simulink model "proprioception_test"  (R2015a)
settings: Solver=ode4  SolverMode=MultiTasking  StartTime=0.0  StopTime=inf  FixedStep=BKIN_STEP_TIME  RelTol=1e-3
StartFcn:
  |  warndlg('Dexterit-E models cannot run under simulation. Please compile your model and run it from within Dexterit-E.');set_param(bdroot,'SimulationCommand','stop')
model workspace (MAT data in the model file):
  col_x = 1
  col_y = 2
  RADIUS_VIS = 3
  COLOR_INIT = 4
  DELAY_POST_TRIAL_COL = 5
  BKIN_STEP_TIME = 0.00025
  COLOR_MOVE = 5
  START_WAIT_TIME_COL = 1
  E_START_TRIAL = 2
  E_START_REACHED = 4
  E_MOVED_EARLY = 21
  E_GO_CUE = 9
  E_MOVE_TIMEOUT = 23
  E_HOLDING_STILL = 12
  E_END_TRIAL = 14
  STROKE_WIDTH = 6
  K_HAND_VEL = 1
  E_MOVE_ON = 10
  K_HOLDTIME = 2
  K_ROBOT_RAMP_TIME = 3
  E_ROBOT_RETURN_TO_START = 33
  E_ENABLED_CONTROLLER = 31
  K_TIME_TO_START = 4
  E_RETURN_TO_START = 35
  E_HOLD_POS = 37
  E_INCREMENTING_TSTEP1 = 6
  E_INCREMENTING_TSTEP2 = 7
  E_INCREMENTING_TSTEP3 = 8
  BKIN_KINEMATIC_FRAME_SIZE = 400
  E_NO_EVENT = 0
  COMP_IS_SAME = 2
  E_QUESTION1 = 40
  REFERENCE_TGT = 6
  CP1 = 7
  CP2 = 8
  CP3 = 9
  CP4 = 10
  MOVE_TO_REF_TIME = 2
  REPOSITION_TIME = 3
  STARTUP_TIME = 4
  COMP_IS_DIFF = 3
  ROTATION = 7
  E_WAIT_JS_THRESH = 16
  E_AT_JS_THRESH = 18
libraries: simulink x5, Video x4, General x3, slrtlib x3, KINARM_loads x2, KINARM_IO x1, KINARM_general x1, xpcnilib x1
CloseFcn:
  | rtwprivate ssgencode ModelCloseRequest b2lab2d
settings Model: ModifiedComment=chris -- Wed Feb 16 09:18:30 2005 -- Version 1.1384  ModifiedHistory=Feb 16/05 - Add error repeat, add offset ramp  ExtModeArmWhenConnect=off  ExtModeLogAll=off  Creator=Chris Grebeldinger  LastModifiedBy=User
settings SolverCC: EnableConcurrentExecution=on  AutoInsertRateTranBlk=on
settings DataIOCC: LimitDataPoints=off  SignalLoggingSaveFormat=ModelDataLogs  SaveOutput=off  SaveTime=off  SignalLoggingName=sigsOut
settings OptimizationCC: BlockReduction=off  BooleanDataType=off  OptimizeBlockIOStorage=off  BufferReuse=off  GlobalBufferReuse=off  ExpressionFolding=off  ExpressionDepthLimit=2147483647  LocalBlockOutputs=off  InitFltsAndDblsToZero=on
settings DebuggingCC: SaveWithParameterizedLinksMsg=none  UnderspecifiedInitializationDetection=Classic  MergeDetectMultiDrivingBlocksExec=none  SignalResolutionControl=TryResolveAllWithWarning  MultiTaskDSMMsg=warning  FcnCallInpInsideContextMsg=UseLocalSettings  StateNameClashWarn=warning  StrictBusMsg=ErrorOnBusTreatedAsVector
settings HardwareCC: ProdIntDivRoundTo=Zero  ProdEndianess=LittleEndian  ProdLongLongMode=on  ProdHWDeviceType=Generic->32-bit x86 compatible  TargetHWDeviceType=32-bit Generic
settings SFSimCC: SimCustomHeaderCode="#include \"stdlib.h\""  SFSimEcho=off  SimParseCustomCode=off
settings RTWCC: SystemTargetFile=slrt.tlc  TemplateMakefile=slrt_default_tmf  Description=Simulink Real-Time  CustomSourceCode="#include \"stdlib.h\""
settings CodeAppCC: MaxIdLength=63
settings SimulinkRealTimeCC: TargetFcnLib=ansi_tfl_tmw.mat  GeneratePreprocessorConditionals=Disable all  xPCisDownloadable=off  xPCisDefaultEnv=off

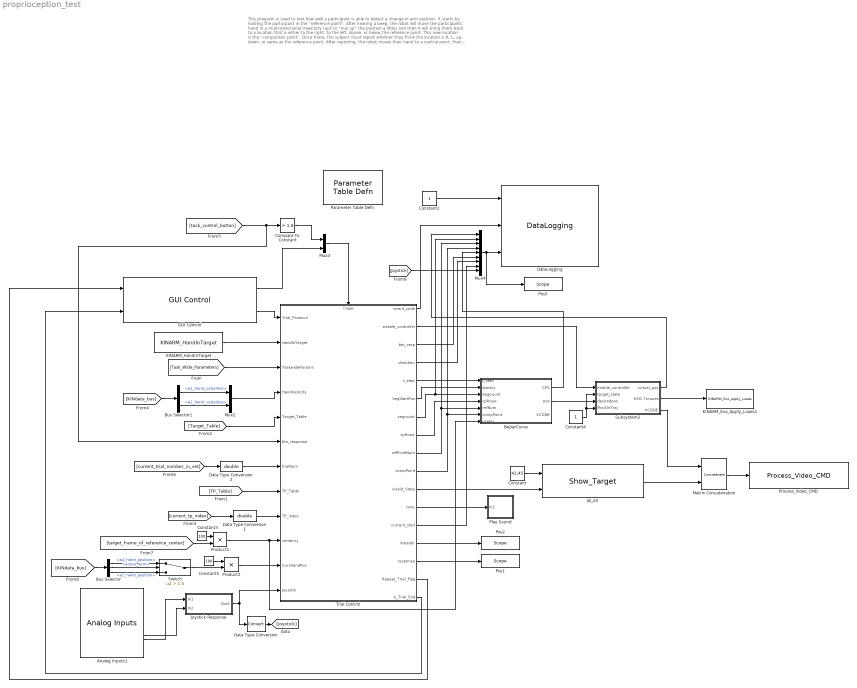
== system proprioception_test ==
  note: This program is used to test how well a participant is able to detect a change in arm position.
      | It starts by holding the participant in the "reference point". After hearing a beep, the robot
      | will move the participants hand in a multi-directional trajectory (just to "mix up" the position a little)
      | and then it will bring them back to a location that is either to the right, to the left, above, or below
      | the reference point. This new location is the "comparison point". Once there, the subject must
      | report whether they think the location is R, L, up, down, or same as the reference point. After
      | reporting, the robot moves their hand to a central point, then back to the reference point to begin
      | the next trial.
      | A staircase updates for each direction, until a direction's staircase experiences 3 duirection
      | reversals in 6 trials, or 25 repetitions.
  Analog Inputs1 : KINARM_IO/Analog Inputs  channel=[1:32]  range=[5, 5, 5, 5, 5, 5, 5, 5,5, 5, 5, 5, 5, 5, 5, 5,5, 5, 5, 5, 5, 5, 5, 5,5, 5, 5, 5, 5, 5, 5, 5,]  coupling=[0, 0, 0, 0, 0, 0, 0, 0,0, 0, 0, 0, 0, 0, 0, 0,0, 0, 0, 0, 0, 0, 0, 0,0, 0, 0, 0, 0, 0, 0, 0,]  scantime6071e=1.28e-5  scantime6229=5e-6  sampletime=0.001  slot=-1  oscantime6071e=0
  BezierCurve : Subsystem
  Bus Selector : BusSelector  OutputSignals=Robot2.a2_hand_position,KINDataGeneral.active_arm,Robot1.a1_hand_position
  Bus Selector1 : BusSelector  OutputSignals=Robot1.a1_hand_velocities,Robot2.a2_hand_velocities
  Compare To Constant : simulink/Logic and Bit Operations/Compare To Constant  relop=>  const=1.0  OutDataTypeStr=boolean
  Constant : Constant  Value=42:45
  Constant2 : Constant
  Constant3 : Constant  Value=100
  Constant4 : Constant
  Constant5 : Constant  Value=100
  Data Type Conversion : DataTypeConversion
  Data Type Conversion1 : DataTypeConversion  OutDataTypeStr=double
  Data Type Conversion2 : DataTypeConversion  OutDataTypeStr=double
  DataLogging : General/DataLogging  log_event_codes=on  log_analog_inputs=on  show_time_remaining=off
  GUI Control : General/GUI Control  target_type_str=Circle  Target_Type=1  XYcols=[1 2]  Vcols=3  Lcols=4  indices_padding=[0 0 0 0;0 0 0 0]  task_version=1.0  show_repeat_trial_flag=on  target_table_rows=64  load_table_rows=20  tp_table_rows=100
  Joystick Response : Subsystem
  KINARM_Exo_Apply_Loads1 : KINARM_loads/KINARM_Exo_Apply_Loads  up_duration=200  down_duration=200  max_torque=6  limit_motors=off
  KINARM_HandInTarget : KINARM_general/KINARM_HandInTarget  use_dominant_hand=on  target_type=Circle  num_states=1  attribcol1=[RADIUS_VIS]  attribcol2=[4]  attribcol3=[5]  attribcol4=[6]  attribcol5=[0]
  Matrix Concatenation : Concatenate  Mode=Multidimensional array
  Mux2 : Mux  Inputs=[2 2]
  Mux3 : Mux  Inputs=2
  Mux4 : Mux  Inputs=9
  Parameter Table Defn : General/Parameter Table Defn  ShowInLibBrowser=0
  Play Sound : Subsystem
  Pos1 : slrtlib/Displays and Logging/Scope   scopeno=2  scopetype=Target  autostart=on  viewmode=Numerical  formatstr='%15.6f'  grid=on  ylimits=[-10,10]  nosamples=250  noprepostsamples=0  interleave=1  triggermode=FreeRun  triggersignal=1  trigsignalfromport=off  triggerlevel=0.0  triggerslope=Either  triggerscope=1  triggersample=0  filename=data.dat  mode=Lazy  writesize=512  autorestart=off  dynamicfilemode=off  maxwritefilesize=512*1024^2
  Pos2 : slrtlib/Displays and Logging/Scope   scopeno=3  scopetype=Target  autostart=on  viewmode=Numerical  formatstr='%15.6f'  grid=on  ylimits=[-10,10]  nosamples=250  noprepostsamples=0  interleave=1  triggermode=FreeRun  triggersignal=1  trigsignalfromport=off  triggerlevel=0.0  triggerslope=Either  triggerscope=1  triggersample=0  filename=data.dat  mode=Lazy  writesize=512  autorestart=off  dynamicfilemode=off  maxwritefilesize=512*1024^2
  Pos5 : slrtlib/Displays and Logging/Scope   scopeno=1  scopetype=Target  autostart=on  viewmode=Numerical  formatstr='%15.6f'  grid=on  ylimits=[-10,10]  nosamples=250  noprepostsamples=0  interleave=1  triggermode=FreeRun  triggersignal=1  trigsignalfromport=off  triggerlevel=0.0  triggerslope=Either  triggerscope=1  triggersample=0  filename=data.dat  mode=Lazy  writesize=512  autorestart=off  dynamicfilemode=off  maxwritefilesize=512*1024^2
  Process_Video_CMD : Video/Process_Video_CMD  video_delay=50
  Product1 : Product
  Product2 : Product
  Subsystem2 : Subsystem
  Switch : Switch  Criteria=u2 > Threshold  Threshold=1.5
  Trial Control : Stateflow chart  TreatAsAtomicUnit=on
  all_dir : Video/Show_Target  target_type=Triangle  num_states=2  attribcol1=[COLOR_INIT 0 0 RADIUS_VIS RADIUS_VIS 0 ROTATION]  attribcol2=[COLOR_MOVE 0 0 RADIUS_VIS RADIUS_VIS 0 ROTATION]  attribcol3=[4 0 0 3 1.5 0 180]  attribcol4=[4 0 0 3 1.5 0 270]  attribcol5=[0 0 24 0 0 0 0]  stateindices_padding=[0 0 0 0;0 0 0 0;0 0 0 0;0 0 0 0;0 0 0 0]  source=dialog  opacity=100  target_display=Both subject and operator displays  num_col=7
  wires:
  [Task_Wide_Parameters] -> Trial Control/3(TaskwideParams)
  Trial Control/1(event_code) -> DataLogging/2
  Mux2/1 -> Trial Control/4(HandVelocity)
  Bus Selector1/1 -> Mux2/1  "<a1_hand_velocities>"
  Bus Selector1/2 -> Mux2/2  "<a2_hand_velocities>"
  [KINdata_bus] -> Bus Selector1/1
  GUI Control/2 -> Trial Control/1(Trial_Protocol)
  [task_control_button] -> Compare To Constant/1, Trial Control/6(btn_response)
  Trial Control/8(cpRows) -> BezierCurve/4(cpRows)
  Trial Control/6(SegStartPos) -> BezierCurve/2(startxy)
  Trial Control/7(segcount) -> Mux4/2, BezierCurve/3(SegCount)
  Trial Control/5(t_step) -> BezierCurve/1(t_step)
  Trial Control/9(refPointNum) -> Mux4/3, BezierCurve/5(refNum)
  BezierCurve/2(pos) -> Subsystem2/3(desiredpos)
  KINARM_HandInTarget/1 -> Trial Control/2(HandInTarget)
  Trial Control/10(compPoint) -> Mux4/4, BezierCurve/6(compPoint)
  Trial Control/12(tone) -> Play Sound/1(In1)
  [Target_Table] -> Trial Control/5(Target_Table)
  Trial Control/16(Repeat_Trial_Flag) -> GUI Control/1
  Mux3/1 -> Trial Control/Trigger
  Mux4/1 -> Pos5/1, DataLogging/3
  Constant2/1 -> DataLogging/1
  Subsystem2/2(EXO Torques) -> KINARM_Exo_Apply_Loads1/1
  Trial Control/17(e_Trial_End) -> GUI Control/2
  GUI Control/1 -> Mux3/2
  Compare To Constant/1 -> Mux3/1
  [TP_Table] -> Trial Control/8(TP_Table)
  [current_tp_index] -> Data Type Conversion1/1
  Data Type Conversion1/1 -> Trial Control/9(TP_index)
  BezierCurve/1(CPS) -> Mux4/5
  Data Type Conversion2/1 -> Trial Control/7(trialNum)
  [current_trial_number_in_set] -> Data Type Conversion2/1
  [target_frame_of_reference_center] -> Product1/2
  Constant3/1 -> Product1/1
  Product1/1 -> Trial Control/10(centerxy), BezierCurve/7(center)
  Trial Control/13(current_stair) -> Mux4/8
  Subsystem2/3(VCODE) -> Matrix Concatenation/1
  Subsystem2/1(virtual_pos) -> Mux4/1
  Constant4/1 -> Subsystem2/2(target_state), Subsystem2/4(MovOnTraj)
  Trial Control/2(enable_controller) -> Subsystem2/1(enable_controller)
  [KINdata_bus] -> Bus Selector/1
  Bus Selector/2 -> Switch/2  "<active_arm>"
  Bus Selector/1 -> Switch/1  "<a2_hand_position>"
  Bus Selector/3 -> Switch/3  "<a1_hand_position>"
  Switch/1 -> Product2/2
  Constant5/1 -> Product2/1
  Product2/1 -> Trial Control/11(CurrHandPos)
  Trial Control/4(direction) -> Mux4/7
  Joystick Response/1(Out1) -> Data Type Conversion/1, Trial Control/12(joystick)
  Trial Control/11(visAid_State) -> all_dir/2
  Constant/1 -> all_dir/1
  all_dir/1 -> Matrix Concatenation/2
  Matrix Concatenation/1 -> Process_Video_CMD/1
  Analog Inputs1/24 -> Joystick Response/1(In1)
  Analog Inputs1/22 -> Joystick Response/2(In2)
  Trial Control/15(response) -> Pos1/1
  Trial Control/14(initialdir) -> Pos2/1
  [joystick] -> Mux4/9
  Trial Control/3(btn_resp) -> Mux4/6
  Data Type Conversion/1 -> [joystick]

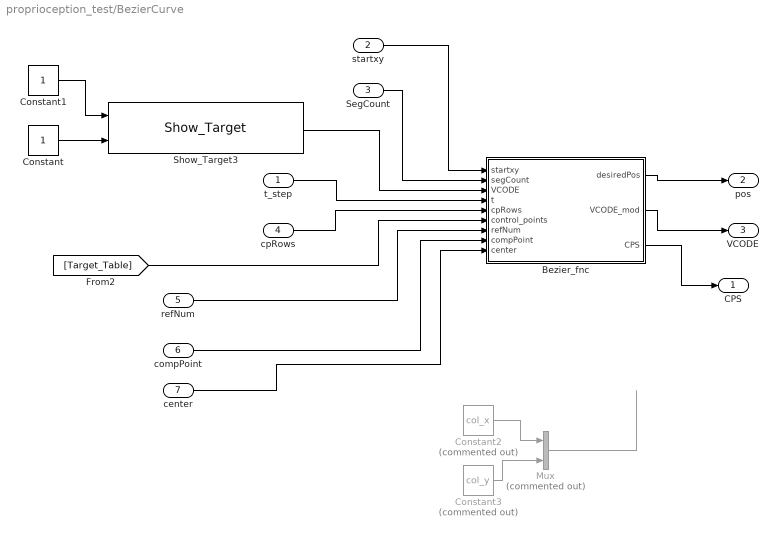
== system proprioception_test/BezierCurve ==
  t_step : Inport  PortDimensions=1
  startxy : Inport  Port=2  PortDimensions=[1 2]
  SegCount : Inport  Port=3  PortDimensions=1
  cpRows : Inport  Port=4  PortDimensions=[1 5]
  refNum : Inport  Port=5  PortDimensions=1
  compPoint : Inport  Port=6  PortDimensions=[1 2]
  center : Inport  Port=7  PortDimensions=[1 2]
  Bezier_fnc : MATLAB Function  TreatAsAtomicUnit=on
  Constant : Constant
  Constant1 : Constant
  Constant2 : Constant  Commented=on  Value=col_x
  Constant3 : Constant  Commented=on  Value=col_y
  Mux : Mux  Commented=on  Inputs=2
  Show_Target3 : Video/Show_Target  target_type=Circle  num_states=1  attribcol1=[COLOR_INIT 0 0 RADIUS_VIS]  attribcol2=[6 6 0 3]  attribcol3=[0 0 0 0]  attribcol4=[0 0 0 0]  attribcol5=[0 0 24 0]  stateindices_padding=[0 0 0 0 0 0 0;0 0 0 0 0 0 0;0 0 0 0 0 0 0;0 0 0 0 0 0 0;0 0 0 0 0 0 0]  source=dialog  opacity=100  target_display=Both subject and operator displays  num_col=4
  CPS : Outport  PortDimensions=[1 8]
  pos : Outport  Port=2  OutDataTypeStr=double  PortDimensions=[1 2]
  VCODE : Outport  Port=3
  wires:
  Show_Target3/1 -> Bezier_fnc/3(VCODE)
  Bezier_fnc/2(VCODE_mod) -> VCODE/1
  [Target_Table] -> Bezier_fnc/6(control_points)
  Bezier_fnc/1(desiredPos) -> pos/1
  Constant1/1 -> Show_Target3/1
  startxy/1 -> Bezier_fnc/1(startxy)
  SegCount/1 -> Bezier_fnc/2(segCount)
  cpRows/1 -> Bezier_fnc/5(cpRows)
  refNum/1 -> Bezier_fnc/7(refNum)
  compPoint/1 -> Bezier_fnc/8(compPoint)
  Constant/1 -> Show_Target3/2
  t_step/1 -> Bezier_fnc/4(t)
  Mux/1 -> ?
  Constant2/1 -> Mux/1
  Constant3/1 -> Mux/2
  Bezier_fnc/3(CPS) -> CPS/1
  center/1 -> Bezier_fnc/9(center)

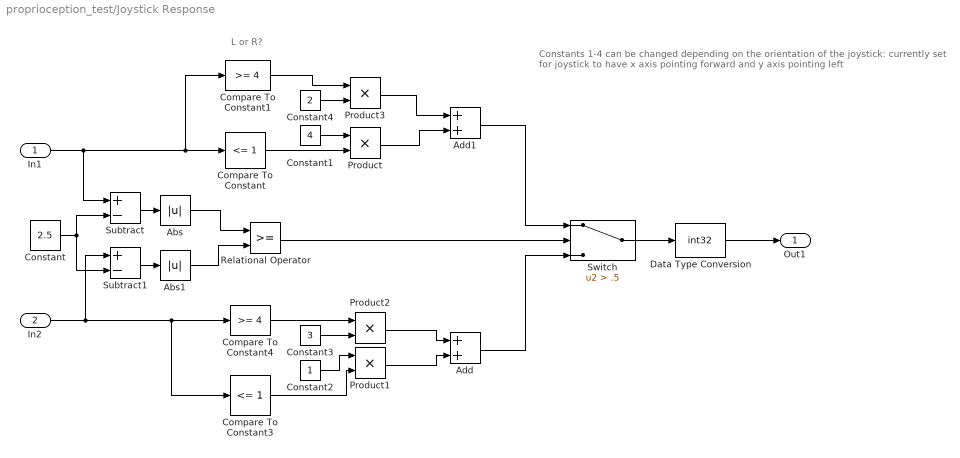
== system proprioception_test/Joystick Response ==
  note: Constants 1-4 can be changed depending on the orientation of the joystick:
      | currently set for joystick to have x axis pointing forward and y axis pointing left
  note: L or R?
  In1 : Inport
  In2 : Inport  Port=2
  Abs : Abs
  Abs1 : Abs
  Add : Sum
  Add1 : Sum
  Compare To Constant : simulink/Logic and Bit Operations/Compare To Constant  relop=<=  const=1  OutDataTypeStr=boolean
  Compare To Constant1 : simulink/Logic and Bit Operations/Compare To Constant  relop=>=  const=4  OutDataTypeStr=boolean
  Compare To Constant3 : simulink/Logic and Bit Operations/Compare To Constant  relop=<=  const=1  OutDataTypeStr=boolean
  Compare To Constant4 : simulink/Logic and Bit Operations/Compare To Constant  relop=>=  const=4  OutDataTypeStr=boolean
  Constant : Constant  Value=2.5
  Constant1 : Constant  Value=4
  Constant2 : Constant
  Constant3 : Constant  Value=3
  Constant4 : Constant  Value=2
  Data Type Conversion : DataTypeConversion  OutDataTypeStr=int32
  Product{,1..3} (4 alike) : Product
  Relational Operator : RelationalOperator  OutDataTypeStr=boolean
  Subtract : Sum  Inputs=+-
  Subtract1 : Sum  Inputs=+-
  Switch : Switch  Criteria=u2 > Threshold  Threshold=.5
  Out1 : Outport
  wires:
  In1/1 -> Subtract/1, Compare To Constant1/1, Compare To Constant/1
  Compare To Constant/1 -> Product/2
  In2/1 -> Subtract1/1, Compare To Constant3/1, Compare To Constant4/1
  Compare To Constant3/1 -> Product1/2
  Compare To Constant4/1 -> Product2/1
  Subtract/1 -> Abs/1
  Subtract1/1 -> Abs1/1
  Constant/1 -> Subtract/2, Subtract1/2
  Abs/1 -> Relational Operator/1
  Abs1/1 -> Relational Operator/2
  Compare To Constant1/1 -> Product3/1
  Constant1/1 -> Product/1
  Constant2/1 -> Product1/1
  Constant3/1 -> Product2/2
  Product2/1 -> Add/1
  Product1/1 -> Add/2
  Product/1 -> Add1/2
  Add1/1 -> Switch/1
  Add/1 -> Switch/3
  Relational Operator/1 -> Switch/2
  Constant4/1 -> Product3/2
  Product3/1 -> Add1/1
  Switch/1 -> Data Type Conversion/1
  Data Type Conversion/1 -> Out1/1

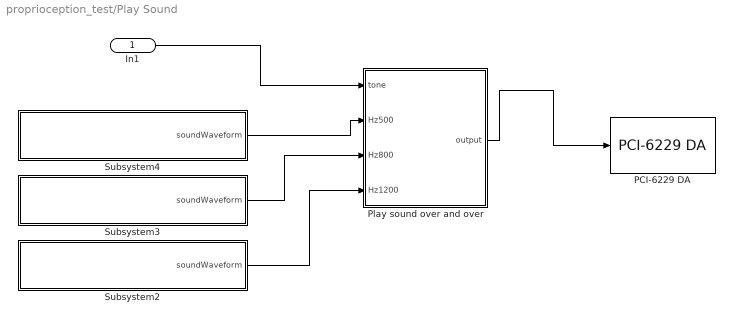
== system proprioception_test/Play Sound ==
  In1 : Inport
  PCI-6229 DA : xpcnilib/D//A/M Series/PCI-6229 DA  channel=[1]  reset=[1]  initValue=[0]  sampletime=-1  slot=-1
  Play sound over and over : MATLAB Function  TreatAsAtomicUnit=on
  Subsystem2 : Subsystem  mask(Load Waveform Into Variable){fileName=Hz1200}
      mask prompts: fileName "Name of .mat Data File (must be in current directory)"
      mask help: This block will load the .MAT file specified in the dialog, and put the first variable into a GoTo called 'soundWaveform'.
      mask init:
      | filenameFromMask = get_param(gcb, 'fileName');
      | 
      | try 
      | 	dataFromFile = load(filenameFromMask);
      | 	names = fieldnames(dataFromFile);
      | 	soundDataFromFile = dataFromFile.(names{1});
      | 	display(['Sound waveform from file ''' filenameFromMask ''' loaded.']);
      | catch ME
      | 	display(ME.message)
      | end
      mask Help:
      | Enter the name a .MAT file containing a single vector or matrix. The .MAT file must be located in the current directory.
      | 
      | The first variable from the .MAT file will be put into a Goto called 'soundWaveform'.
      mask Display: disp(['Load waveform from ''' filenameFromMask ''''])
  Subsystem3 : Subsystem  mask(Load Waveform Into Variable){fileName=Hz800}
      mask prompts: fileName "Name of .mat Data File (must be in current directory)"
      mask help: This block will load the .MAT file specified in the dialog, and put the first variable into a GoTo called 'soundWaveform'.
      mask init: same as proprioception_test/Play Sound/Subsystem2
      mask Help:
      | Enter the name a .MAT file containing a single vector or matrix. The .MAT file must be located in the current directory.
      | 
      | The first variable from the .MAT file will be put into a Goto called 'soundWaveform'.
      mask Display: disp(['Load waveform from ''' filenameFromMask ''''])
  Subsystem4 : Subsystem  mask(Load Waveform Into Variable){fileName=Hz500}
      mask prompts: fileName "Name of .mat Data File (must be in current directory)"
      mask help: This block will load the .MAT file specified in the dialog, and put the first variable into a GoTo called 'soundWaveform'.
      mask init: same as proprioception_test/Play Sound/Subsystem2
      mask Help:
      | Enter the name a .MAT file containing a single vector or matrix. The .MAT file must be located in the current directory.
      | 
      | The first variable from the .MAT file will be put into a Goto called 'soundWaveform'.
      mask Display: disp(['Load waveform from ''' filenameFromMask ''''])
  wires:
  Play sound over and over/1(output) -> PCI-6229 DA/1
  Subsystem3/1(soundWaveform) -> Play sound over and over/3(Hz800)
  Subsystem4/1(soundWaveform) -> Play sound over and over/2(Hz500)
  In1/1 -> Play sound over and over/1(tone)
  Subsystem2/1(soundWaveform) -> Play sound over and over/4(Hz1200)

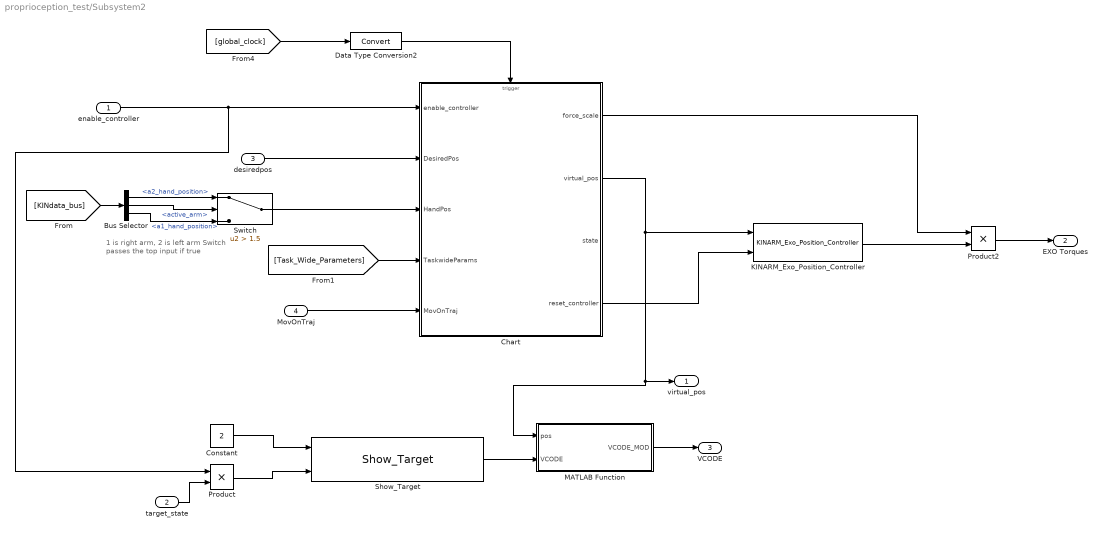
== system proprioception_test/Subsystem2 ==
  note: 1 is right arm, 2 is left arm
      | Switch passes the top input if true
  enable_controller : Inport
  target_state : Inport  Port=2
  desiredpos : Inport  Port=3
  MovOnTraj : Inport  Port=4
  Bus Selector : BusSelector  OutputSignals=Robot2.a2_hand_position,KINDataGeneral.active_arm,Robot1.a1_hand_position
  Chart : Stateflow chart  TreatAsAtomicUnit=on
  Constant : Constant  Value=2
  Data Type Conversion2 : DataTypeConversion
  KINARM_Exo_Position_Controller : KINARM_loads/KINARM_Exo_Position_Controller  use_dom_hand=on  KINARM_Type=Human  inertias_for_FF=KINARM robot & arm troughs & subject  angles_or_XY=End-point (global x/y)  sample_time=0.001
  MATLAB Function : MATLAB Function  TreatAsAtomicUnit=on
  Product : Product
  Product2 : Product
  Show_Target : Video/Show_Target  target_type=Circle  num_states=1  attribcol1=[COLOR_INIT 0 0 RADIUS_VIS]  attribcol2=[6 6 0 3]  attribcol3=[0 0 0 0]  attribcol4=[0 0 0 0]  attribcol5=[0 0 24 0]  stateindices_padding=[0 0 0 0 0 0 0;0 0 0 0 0 0 0;0 0 0 0 0 0 0;0 0 0 0 0 0 0;0 0 0 0 0 0 0]  source=dialog  opacity=100  target_display=Both subject and operator displays  num_col=4
  Switch : Switch  Criteria=u2 > Threshold  Threshold=1.5
  virtual_pos : Outport
  EXO Torques : Outport  Port=2
  VCODE : Outport  Port=3
  wires:
  [KINdata_bus] -> Bus Selector/1
  Bus Selector/2 -> Switch/2  "<active_arm>"
  [Task_Wide_Parameters] -> Chart/4(TaskwideParams)
  [global_clock] -> Data Type Conversion2/1
  Data Type Conversion2/1 -> Chart/Trigger
  Chart/2(virtual_pos) -> MATLAB Function/1(pos), virtual_pos/1, KINARM_Exo_Position_Controller/1
  MovOnTraj/1 -> Chart/5(MovOnTraj)
  Switch/1 -> Chart/3(HandPos)
  desiredpos/1 -> Chart/2(DesiredPos)
  Constant/1 -> Show_Target/1
  Show_Target/1 -> MATLAB Function/2(VCODE)
  MATLAB Function/1(VCODE_MOD) -> VCODE/1
  KINARM_Exo_Position_Controller/1 -> Product2/2
  Product2/1 -> EXO Torques/1
  Chart/1(force_scale) -> Product2/1
  Chart/4(reset_controller) -> KINARM_Exo_Position_Controller/2
  Bus Selector/1 -> Switch/1  "<a2_hand_position>"
  Bus Selector/3 -> Switch/3  "<a1_hand_position>"
  enable_controller/1 -> Product/1, Chart/1(enable_controller)
  Product/1 -> Show_Target/2
  target_state/1 -> Product/2

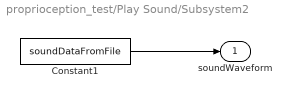
== system proprioception_test/Play Sound/Subsystem2 ==
  Constant1 : Constant  Value=soundDataFromFile  SampleTime=-1
  soundWaveform : Outport
  wires:
  Constant1/1 -> soundWaveform/1

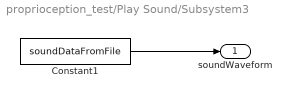
== system proprioception_test/Play Sound/Subsystem3 ==
  Constant1 : Constant  Value=soundDataFromFile
  soundWaveform : Outport
  wires:
  Constant1/1 -> soundWaveform/1

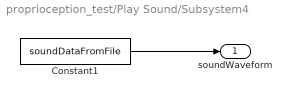
== system proprioception_test/Play Sound/Subsystem4 ==
  Constant1 : Constant  Value=soundDataFromFile
  soundWaveform : Outport
  wires:
  Constant1/1 -> soundWaveform/1

== matlab function proprioception_test/Play Sound/Play sound over and over ==
  data: tone input; output output; Hz500 input; Hz800 input; Hz1200 input
function output = fcn(tone,Hz500,Hz800,Hz1200)
%#codegen

persistent t last_tone_state
if isempty(t), t = 0; end
if isempty(last_tone_state), last_tone_state = 0; end

trigger = last_tone_state ~= tone;
if trigger > 0
    last_tone_state = tone;
end

output = 0;		% default
if t == 0 && trigger > 0
	% start the playing of the sound.
	t = t + 1;
end

if tone == 1
    data = Hz500;
elseif tone == 2
    data = Hz800;
elseif tone == 3
    data = Hz1200;
else 
    t = 0;
    data = 0;
end

if t > 0
	output = data(t);
	if t == length(data)
		t = 0;
	else
		t = t + 1;
	end
end

== stateflow chart proprioception_test/Trial Control ==
  note: ?
  state Initialize/
    //Initialization state
    Repeat_Trial_Flag = 0;
    ramp_time = TaskwideParams[K_ROBOT_RAMP_TIME];
    enable_controller = 0;
    tone = 0;
    segcount = -1;
    response = 0;
    initialdir = 0;
    currentdir = 0;
    visAid_State[1] = 0;visAid_State[2] = 0;visAid_State[3] = 0;visAid_State[4] = 0;
    last_refPointNum = 0;
    direction = 0;
    [distances,staircases,NoticedIncorrect,finished,refPointsFinished] = init_vars();
    current_stair = distances;
  state MainTrial
    state ChooseCompPoint/
      direction = ceil((rand()/single(RAND_MAX))*4);
      refPointNum = Trial_Protocol[REFERENCE_TGT];
      old_finished = finished;
      stairNum = direction + (refPointNum-1)*4;
      [nFinished, refPointsFinished,finished] = findFinished(old_finished,staircases,stairNum);
      Repeat_Trial_Flag = 0;
      btn_resp = 0;
    state OneRefPointFinished3/
      //skip over it
      Repeat_Trial_Flag = 0;
      enable_controller = 0;
    state MoveToOrigin/
      event_code = E_START_TRIAL;
      SegStartPos[1] = compPoint[1];
      SegStartPos[2] = compPoint[2];
      event_code = E_START_REACHED;
      tickCount = Trial_Protocol[START_WAIT_TIME_COL] ;
      segcount = 4;
      t_step = 0;
      //increment t_step on each clock cycle
      during:
      on e_clk: t_step = t_step + (1/ (Trial_Protocol[MOVE_TO_REF_TIME]/1000 * 1000));
    state FirstTrial_Seg1/
      //from origin, move to new reference point
      enable_controller = 1;
      event_code = E_START_TRIAL;
      refPointPos[1] = Target_Table[refPointNum][1];
      refPointPos[2] = Target_Table[refPointNum][2];
      segcount = 1;
      SegStartPos[1] = CurrHandPos[1];
      SegStartPos[2] = CurrHandPos[2];
      t_step = 0;
      during:
      on e_clk: t_step = t_step +  (1/(Trial_Protocol[STARTUP_TIME]/1000 * 1000));
    state MoveToReference_Seg1/
      //from origin, move to new reference point
      event_code = E_START_TRIAL;
      refPointPos[1] = Target_Table[refPointNum][1];
      refPointPos[2] = Target_Table[refPointNum][2];
      event_code = E_START_REACHED;
      tickCount = Trial_Protocol[START_WAIT_TIME_COL] ;
      segcount = 1;
      SegStartPos[1] = centerxy[1]-12;
      SegStartPos[2] = centerxy[2]+18;
      t_step = 0;
      //increment t_step on each clock cycle
      during:
      on e_clk: t_step = t_step + (1/ (Trial_Protocol[MOVE_TO_REF_TIME]/1000 * 1000));
    state OneRefPointFinished4/
      tone = 1;
      tickCount = Trial_Protocol[START_WAIT_TIME_COL] ;
    state wait/
      tickCount = 200;
    state Reposition_Seg2/
      // The hand is in the reference point so start respositioning it by incrementing t_step
      event_code = E_INCREMENTING_TSTEP1;
      cpRows[1] = Trial_Protocol[CP1]; //CP1
      cpRows[2] = Trial_Protocol[CP2];
      cpRows[3] =  Trial_Protocol[CP3];
      cpRows[4] =  Trial_Protocol[CP4];//CP4
      [compPoint[1],compPoint[2]] = findComparisonPoint(distances[1][stairNum],refPointPos,direction);
      segcount = 2;
      SegStartPos = refPointPos;
      t_step = 0;
      during:
      on e_clk: t_step = t_step + (1/ (Trial_Protocol[REPOSITION_TIME]/1000 * 1000));
    state wait1/
      tickCount = 200;
    state WaitForReport/
      //hold hand in the comparison and wait for the subject to report same or different
      tone = 2;
      event_code = E_QUESTION1;
    state CheckResp/
      btn_resp = btn_response;
      response = 0;
    state TimeAtThresh/
      event_code = E_AT_JS_THRESH;
      tickCount = 1500;
    state WaitForThreshold/
      event_code = E_WAIT_JS_THRESH;
      visAid_State[1] =1; visAid_State[2] =1;
      visAid_State[3] =1; visAid_State[4] =1;
      response = joystick;
      during:
      response = joystick;
    state EndOfTrialChanges/
      //record what ref point was used, change current values to old values since trial proceeded
      old_distances = distances;
      old_staircases = staircases;
      old_finished = finished;
      old_NoticedIncorrect = NoticedIncorrect;
      last_refPointNum = refPointNum;  //for comparison to the next choice of ref Point
      [finished, distances, staircases, NoticedIncorrect] = update_stairs(response,direction,last_refPointNum,old_distances,...
      old_staircases,old_finished,old_NoticedIncorrect,trialNum);
      current_stair = distances; // send this to the analog inputs
      tickCount = Trial_Protocol[DELAY_POST_TRIAL_COL];
    state EndOfTrial/
      //record what ref point was used, reset values
      event_code = E_END_TRIAL;
    (junction 249) -> OneRefPointFinished3 [order 4] : //experiment is over
        | [nFinished == 1 || trialNum == 100]
    (junction 249) -> ChooseCompPoint [order 1] : //has this direction finished? (but not the entire ref point?)
        | [finished[stairNum] == 1 && refPointsFinished[refPointNum]~=1]
    OneRefPointFinished3 -> EndOfTrial
    ChooseCompPoint -> (junction 249)
    (junction 249) -> MoveToOrigin [order 2] : //continue if staircase is unfinished (and not a repeat) and not the first trial
        | [finished[stairNum] == 0 && trialNum ~=1]
    (junction 249) -> FirstTrial_Seg1 [order 3] : //1st trial?
        | [trialNum == 1]
    MoveToOrigin -> MoveToReference_Seg1 : // hand at arbitrary point
        | [(t_step >= 1)]/
        | t_step = 1;
    MoveToReference_Seg1 -> wait : // t done incrementing
        | [(t_step >= 1)]/
        | t_step = 1;
    FirstTrial_Seg1 -> wait : // t done incrementing
        | [(t_step >= 1)]/
        | t_step = 1;
    wait -> OneRefPointFinished4 : after(tickCount,e_clk)
    OneRefPointFinished4 -> Reposition_Seg2 : // wait in reference point
        | after(tickCount,e_clk)
    Reposition_Seg2 -> wait1 : [(t_step >= 1)]/
        | t_step = 1;
    wait1 -> WaitForReport : after(tickCount,e_clk)
    WaitForReport -> CheckResp : e_resp_btn/
        | event_code = 50;
    CheckResp -> WaitForThreshold [order 2] : [btn_response == 3]/
    CheckResp -> EndOfTrialChanges [order 1] : [btn_response == 2]/
        | response = 0;
    WaitForThreshold -> TimeAtThresh : [after(1,e_clk) && (response ~= 0)]/
        | visAid_State[response] = 2;
        | //only happens if past thresh
    TimeAtThresh -> WaitForThreshold [order 2] : [after(1,e_clk) && (joystick < 1  || response ~= joystick)]/
        | visAid_State[response] = 1;
        | response = 0;
    TimeAtThresh -> EndOfTrialChanges [order 1] : [after(tickCount,e_clk)]/
        | visAid_State[1] =0; visAid_State[2] =0;
        | visAid_State[3] =0; visAid_State[4] =0;
    EndOfTrialChanges -> EndOfTrial
  note: ?
  state Inter_Trial_State/
    //reset the event code, and send the
    //e_Trial_End Stateflow event to indicate that the trial is over.
    event_code = 0;
    tickCount = Trial_Protocol[DELAY_POST_TRIAL_COL]
    e_Trial_End;
  state RobotRampDown/
    enable_controller = 0;
    ramp_time = 2000;
  (default) -> Initialize
  Initialize -> ChooseCompPoint
  Inter_Trial_State -> ChooseCompPoint : // has a a specified period of
      | // time occured?
      | after(tickCount, e_clk)
  MainTrial -> RobotRampDown : e_ExitTrialNow/
      | tickCount = 1;
      | // e_ExitTrialNow event occurs if the
      | // Dex pause is pressed by the operator
  RobotRampDown -> Inter_Trial_State : after(ramp_time,e_clk)
  EndOfTrial -> Inter_Trial_State : after(tickCount, e_clk)
  data: distFromStaircase function_input double; RefPointPosition function_input double size=[1 2]; stepdir function_input double; x function_output double; y function_output double; oldFinished function_input double size=[1 8]; in_staircases function_input double size=[300 8]; stairNumber function_input double; numFinished function_output double size=1; fin temporary double size=[1 2]; refPtsFinished function_output double size=[1 2]; is_finished function_output double size=[1 8]; dists function_output double size=[1 8]; stairs function_output double size=[300 8]; Noticed_Incorrect function_output double size=[1 8]; is_finished function_output double size=[1 8]; refPtsFinished function_output double size=[1 2]; is_finished function_output double size=[1 8]; dists function_output double size=[1 8]; resp function_input double size=1; dir function_input double size=1; refPtNum function_input double size=1; oldDistances function_input double size=[1 8]; oldStaircases function_input double size=[300 8]; oldFinished function_input double size=[1 8]; stairs function_output double size=[300 8]; oldNoticedIncorrect function_input double size=[1 8]; Noticed_Incorrect function_output double size=[1 8]; trNum function_input double size=1; data local double; elapsed_time local double; event_code output uint16 [0..] =0; enable_controller output double; btn_resp output double; direction output double; tickCount local double; Trial_Protocol input double; HandInTarget input double; TaskwideParams input double; HandVelocity input double; ramp_time local double; t_step output double size=1; SegStartPos output double size=[1 2]; segcount output double size=1; cpRows output double size=[1 5]; refPointNum output double size=1; compPoint output double size=[1 2]; visAid_State output double size=[1 4]; Target_Table input double size=[64 25]; btn_response input double size=1; trialNum input double size=1; distances local double size=[1 8]; staircases local double size=[300 8]; NoticedIncorrect local double size=[1 8]; old_distances local double size=[1 8]; old_staircases local double size=[300 8]; finished local double size=[1 8]; old_finished local double size=[1 8]; old_NoticedIncorrect local double size=[1 8]; refPointPos local double size=[1 2]; refPointsFinished local double size=[1 2]; last_refPointNum local double size=1; nFinished local double; TP_Table input double size=[100 50]; TP_index input double size=1; centerxy input double size=[1 2]; tone output double size=1; current_stair output double size=[1 8]; stairNum local double; CurrHandPos input double size=[1 2]; joystick input int32 size=1; initialdir output double size=1; response output double size=1; Repeat_Trial_Flag output boolean; currentdir local double
  events: e_resp_btn input EITHER_EDGE_EVENT; e_clk input RISING_EDGE_EVENT; e_ExitTrialNow input EITHER_EDGE_EVENT; e_Trial_End output EITHER_EDGE_EVENT
  function [x,y]  = findComparisonPoint(distFromStaircase,RefPointPosition,stepdir):
    | function [x,y]  = findComparisonPoint(distFromStaircase,RefPointPosition,stepdir)
    | 
    | %find the index to the last control point in the TP table
    | 
    | if stepdir == 1   %right
    |     Dir = [1 0];
    | elseif stepdir == 2   %up
    |     Dir = [0 1];    
    | elseif stepdir == 3   %Left
    |     Dir = [-1 0];    
    | elseif stepdir == 4   %down
    |     Dir = [0 -1];
    | else
    |     Dir = [0 0];
    | end
    | 
    | x = RefPointPosition(1,1) + Dir(1)*distFromStaircase;
    | y = RefPointPosition(1,2) + Dir(2)*distFromStaircase;
  function [numFinished, refPtsFinished,is_finished] = findFinished(oldFinished,in_staircases,stairNumber):
    | function [numFinished, refPtsFinished,is_finished] = findFinished(oldFinished,in_staircases,stairNumber)
    | 
    | fin = [0 0];
    | 
    | history = nonzeros(in_staircases(:,stairNumber));
    | is_finished = oldFinished;
    | if length(history) >= 25
    |     is_finished(stairNumber) = 1;
    | end
    | 
    | fin(1) = sum(is_finished(1:4))/4;
    | fin(2) = sum(is_finished(5:8))/4;
    | 
    | numFinished = sum(fin==1);
    | refPtsFinished = [0 0];
    | if fin(1) == 1 
    |     refPtsFinished(1) = 1;
    | else 
    |     refPtsFinished(1) = 0;
    | end
    | if fin(2) == 1   
    |     refPtsFinished(2) = 1;
    | else 
    |     refPtsFinished(2) = 0;
    | end
    | 
    | %check for 25 trials done
  function [dists,stairs,Noticed_Incorrect,is_finished,refPtsFinished] = init_vars:
    | function [dists,stairs,Noticed_Incorrect,is_finished,refPtsFinished] = init_vars()
    | 
    | %'staircases' = 12 columns.  Each column represents a comparison point.
    | %starting with to the right of the first reference point, then above the
    | %1st reference point ... ending with below the last reference point 
    | 
    | %first row of 'staircases' = distance
    | %second row = number of times noticed difference but incorrecet direction
    | 
    | % for aa = 1:12
    | %     if rand>.5
    | %         distances(aa) = .01;
    | %     else 
    | %         distances(aa) = 5;
    | %     end
    | % end
    | dists = [10 10 .5 .5 .5 .5 10 10];
    | refPtsFinished = [0 0];
    | is_finished = zeros(1,8);
    | Noticed_Incorrect = zeros(1,8);
    | stairs = zeros(300,8);
    | stairs(1,:) = dists;
  function [is_finished,dists,stairs,Noticed_Incorrect]   = update_stairs(resp,...:
    | function [is_finished,dists,stairs,Noticed_Incorrect]   = update_stairs(resp,...
    |     dir,refPtNum,oldDistances,oldStaircases,oldFinished,oldNoticedIncorrect,trNum)
    | 
    | %'staircases' = 12 columns.  Each column represents a comparison point.
    | %starting with to the right of the first reference point, then above the
    | %1st reference point ... ending with below the last reference point 
    | %first row of 'staircases' = distance
    | %second row = number of reversals for corresponding comparison point
    | %third row = number of times noticed difference but incorrecet direction
    | 
    | %FOR RESPONSES
    | % 2 = same
    | % 3 = right
    | % 4 = above 
    | % 5 = up 
    | % 6 = left
    | % 7 = below
    | 
    | stairNum = dir + (refPtNum-1)*4; %index for the stair to change
    | new_distances = oldDistances;
    | is_finished = oldFinished;
    | Noticed_Incorrect = oldNoticedIncorrect;
    | stairs = oldStaircases;
    | 
    | %check for reversals
    | reversals = 0;
    | if length(nonzeros(stairs(:,stairNum))) > 8 %only check if one comppoint has been used more than 6 times
    |     history = nonzeros(stairs(:,stairNum));
    |     trend = diff(history);
    |     for a = 6:-1:0 %check the last 7 trials
    |         if trend(end-a)*trend(end-a-1) < 0
    |             reversals = reversals + 1;
    |         end
    |     end
    | end
    | 
    | %clear reversals if at floor
    | if stairs(stairNum) <= .5
    |     reversals = 0;
    | end
    | 
    | %direction is finished if > 3 reversals
    | if reversals >= 3
    |     is_finished(stairNum) = 1;
    | end
    | 
    | 
    | %check total reversals
    | nrevs = 0;
    | history = nonzeros(stairs(:,stairNum));
    | trend = diff(history);
    | if length(trend) > 2
    |     for a = 2:length(trend) %check num reversals in total (if >1 , change step size to .5)
    |         if trend(a)*trend(a-1) < 0
    |             nrevs = nrevs+1;
    |         end
    |     end
    | end
    | 
    | %% update distances
    | 
    | if  resp == 0 %incorrect.
    |     %step up
    |     new_distances(stairNum) = oldDistances(stairNum)+.5;
    |     Noticed_Incorrect(stairNum) = 0;
    | 
    | elseif resp == dir   %correct!
    |     %step down
    |     if length(history) <= 1
    |         new_distances(stairNum) = oldDistances(stairNum)-2;
    |     elseif nrevs < 1  && history(1) == 10 %once one reversal has occurred step by .5 or if started at the bottom step
    |         new_distances(stairNum) = oldDistances(stairNum)-1;
    |     else
    |         new_distances(stairNum) = oldDistances(stairNum)-.5;
    |     end
    |     Noticed_Incorrect(stairNum) = 0;
    |     
    | else   %noticed the difference but not in the right direction
    |     Noticed_Incorrect(stairNum) = oldNoticedIncorrect(stairNum)+1;
    |     if Noticed_Incorrect(stairNum) >= 3  %if this happens 3 times in a row
    |         %step down
    |         new_distances(stairNum) = oldDistances(stairNum)-.5;
    |     end
    | end
    | 
    | %these are the new distances for each compPoint (only one should change each time this fxn is called)
    | dists = new_distances;
    | dists(dists < .5) = .5;
    | new_stair = dists(stairNum); %what we will add to the "staircases" variable below
    | stairs(trNum,stairNum) = new_stair;

== matlab function proprioception_test/BezierCurve/Bezier_fnc ==
  data: startxy input size=[1 2]; segCount input; desiredPos output size=[1 2]; VCODE input; VCODE_mod output; t input; cpRows input size=[1 5]; control_points input; refNum input; compPoint input size=[1 2]; CPS output size=[1 8]; center input
function [desiredPos,VCODE_mod, CPS] = fcn(startxy,segCount,VCODE,t,cpRows,control_points,refNum,compPoint,center)
%#codegen

VCODE_mod = VCODE;

%clip t just in case!
if t < 0
    t = 0;
elseif t > 1;
    t = 1;
end

t = t-sin(2*pi*t)/(2*pi);  %use the bell-shaped velocity profile from the trajectory controller

dPos = [0 0];
cp1 = [0 0];
cp2 = [0 0];
cp3 = [0 0];
cp4 = [0 0];
cp5 = [0 0];
cp6 = [0 0];

% first seg is always used to get the hand to the next trial's reference
if segCount == 1
    %linear bezier using origin and reference
    %point from the next trial
    cp1 = startxy;
    cp2 = [control_points(refNum,1), control_points(refNum,2)];
    cp3 = [NaN NaN];
    cp4 = [NaN NaN];
    cp5 = [NaN NaN];
    
    dPos = (1-t)*cp1 + t*cp2;

elseif segCount == 2 
    %cubic bezier starts at reference
    cp1 = startxy;
    cp2 = [control_points(cpRows(1),1)+startxy(1)-center(1), control_points(cpRows(1),2)+startxy(2)-center(2)]; %CP1X and CP1Y
    cp3 = [control_points(cpRows(2),1)+startxy(1)-center(1), control_points(cpRows(2),2)+startxy(2)-center(2)]; %CP2X and CP2Y
    cp4 = [control_points(cpRows(3),1)+startxy(1)-center(1), control_points(cpRows(3),2)+startxy(2)-center(2)]; %CP3X and CP3Y
    cp5 = [control_points(cpRows(4),1)+startxy(1)-center(1), control_points(cpRows(4),2)+startxy(2)-center(2)]; %CP4X and CP4Y
    cp6 = compPoint;
    
    dPos = ((1-t)^5)*cp1 + 5*t*((1-t)^4)*cp2 + 10*(t^2)*((1-t)^3)*cp3 + 10*(t^3)*((1-t)^2)*cp4 + 5*(t^4)*(1-t)*cp5 + (t^5)*cp6;

elseif segCount == 4
    cp1 = compPoint;%[startxy(1) startxy(2)];
    cp2 = [center(1)-12 center(2)+18];  %this is the reset point
    cp3 = [NaN NaN];
    cp4 = [NaN NaN];
    cp5 = [NaN NaN];

    dPos = (1-t)*cp1 + t*cp2;
    
else    
    cp1 = [NaN NaN];
    cp2 = [NaN NaN];
    cp3 = [NaN NaN];
    cp4 = [NaN NaN];
    cp5 = [NaN NaN];
    
    dPos = startxy;
end



desiredPos = dPos; %to get to cm
desiredPos = desiredPos/100;

CPS = [cp2 cp3 cp4 cp5];

VCODE_mod(3) = desiredPos(1); %convert to meters
VCODE_mod(4) = desiredPos(2); %convert to meters

% elseif segCount == 3 
%     %cubic ends at compPoint
%     cp1 = [control_points(cpRows(3),1), control_points(cpRows(3),2)];
%     cp2 = [control_points(cpRows(4),1), control_points(cpRows(4),2)]; %CP4X and CP4Y
%     cp3 = [control_points(cpRows(5),1), control_points(cpRows(5),2)];
%     cp4 = compPoint;
%     
%     dPos = ((1-t)^3)*cp1 + 3*((1-t)^2)*t*cp2 + 3*(1-t)*(t^2)*cp3 + (t^3)*cp4;

== stateflow chart proprioception_test/Subsystem2/Chart ==
  state EnableState/
    state AutoMoveToPos/
      //smoothly creates a trajectory to get the hand to a point eventually
      state MovingToDesiredXY/
        tickCount = TaskwideParams[K_TIME_TO_START];
        state = 11;
        tick = 0;
        during:
        on e_clk: tick++;
        // the trajectory velocity will have a bell shaped profile
        trajectory_shape = tick/tickCount-sin(2*pi*tick/tickCount)/(2*pi);
        virtual_pos[1] = StartPos[1] + (TgtPos[1] - StartPos[1]) * trajectory_shape;
        virtual_pos[2] = StartPos[2] + (TgtPos[2] - StartPos[2]) * trajectory_shape;
      state GetDesiredXY/
        //grab the current desired pos in case it changes
        TgtPos[1] = DesiredPos[1];
        TgtPos[2] = DesiredPos[2];
        StartPos[1] = HandPos[1];
        StartPos[2] = HandPos[2];
        updatepos = 0;
        state = 10;
      state HoldAtDesiredXY/
        //pause until something changes
        state = 12;
        updatepos = 0;
        during:
        on e_clk: updatepos = ( (abs(TgtPos[1]-DesiredPos[1]) > 0.01) || (abs(TgtPos[2]-DesiredPos[2]) > 0.01) )
      GetDesiredXY -> MovingToDesiredXY : after(1, e_clk)
      HoldAtDesiredXY -> GetDesiredXY : [updatepos == 1 && MovOnTraj == 0]
      MovingToDesiredXY -> HoldAtDesiredXY : after(tickCount, e_clk)/
    state MoveAlongTraj/
      //take a step along a trajectory specified externally
      state GetDesiredXY_Traj/
        TgtPos[1] = DesiredPos[1];
        TgtPos[2] = DesiredPos[2];
        StartPos[1] = HandPos[1];
        StartPos[2] = HandPos[2];
        state = 21;
        //movIsSafe = ( (abs(TgtPos[1]-HandPos[1]) < 0.02) || (abs(TgtPos[2]-HandPos[2]) < 0.02) );
        movIsSafe = 1;
      state MovAlongTraj/
        state = 22;
        virtual_pos[1] = DesiredPos[1];
        virtual_pos[2] = DesiredPos[2];
      GetDesiredXY_Traj -> MovAlongTraj [order 2] : [movIsSafe == 1]
      MovAlongTraj -> GetDesiredXY_Traj
    (junction 15) -> GetDesiredXY [order 1] : [MovOnTraj == 0]
    (junction 15) -> GetDesiredXY_Traj [order 2] : [MovOnTraj == 1]
    MoveAlongTraj -> GetDesiredXY : [MovOnTraj == 0]
    GetDesiredXY_Traj -> GetDesiredXY [order 1] : [movIsSafe == 0]
    AutoMoveToPos -> GetDesiredXY_Traj : [MovOnTraj == 1]
  state Init/
    ramp_time = TaskwideParams[K_ROBOT_RAMP_TIME];
    scale_increment = 1/ramp_time;
    force_scale = 0;
    state = 1;
    during:
    CurHandPos[1] = HandPos[1];
    CurHandPos[2] = HandPos[2];
  state RampUp/
    //ramp up the force scale to 1
    CurHandPos[1] = HandPos[1];
    CurHandPos[2] = HandPos[2];
    virtual_pos[1] = HandPos[1];
    virtual_pos[2] = HandPos[2];
    state = 2;
    force_scale = 0;
    during:
    on e_clk: force_scale += scale_increment;
  state ResetController/
    reset_controller;
  state RampDown/
    //ramp down the force scale to 1
    CurHandPos[1] = HandPos[1];
    CurHandPos[2] = HandPos[2];
    virtual_pos[1] = CurHandPos[1];
    virtual_pos[2] = CurHandPos[2];
    state = 30
    during:
    on e_clk: force_scale -= scale_increment;
  (default) -> Init
  Init -> ResetController : //if controller becomes enabled
      | [enable_controller == 1]/
      | force_scale = 0;
  ResetController -> RampUp
  RampUp -> (junction 15) [order 2] : [force_scale >= 1]/
      | force_scale = 1;
  RampDown -> Init [order 2] : [force_scale <0]/
      | force_scale = 0;
  RampDown -> RampUp [order 1] : [enable_controller == 1]
      | //if the controller is enabled
  RampUp -> RampDown [order 1] : [enable_controller == 0]
      | //if the controller gets shut off
  EnableState -> RampDown : [enable_controller == 0]
  data: enable_controller input double; DesiredPos input; HandPos input; TaskwideParams input; force_scale output double; virtual_pos output double size=2; tickCount local double; StartPos local double size=2; TgtPos local double size=2; updatepos local boolean; MovOnTraj input double; CurHandPos local double size=2; ramp_time local double; scale_increment local double; tick local double; trajectory_shape local double; movIsSafe local boolean; pi constant double =3.14159265358979; state output double
  events: e_clk input EITHER_EDGE_EVENT; reset_controller output EITHER_EDGE_EVENT

== matlab function proprioception_test/Subsystem2/MATLAB Function ==
  data: pos input; VCODE_MOD output; VCODE input
function VCODE_MOD = fcn(pos,VCODE)
%#codegen

VCODE_MOD = VCODE;

VCODE_MOD(3) = pos(1);
VCODE_MOD(4) = pos(2);
